simulink model "STP"  (R2021b)
settings: Solver=VariableStepAuto  StartTime=0.0  StopTime=20  RelTol=1e-3
values from neighbouring files (symbols this model uses):
  a0 = mianownik_d(1,4)    [StpProjekt1.m]
  a1 = mianownik_d(1,3)    [StpProjekt1.m]
  a2 = mianownik_d(1,2)    [StpProjekt1.m]
  b0 = licznik_d(1,4)    [StpProjekt1.m]
  b1 = licznik_d(1,3)    [StpProjekt1.m]
  b2 = licznik_d(1,2)    [StpProjekt1.m]
  K_zr = acker(AII,BII,[zb zb zb])    [StpProjekt1.m]
  L1 = acker(A',C', [zo1 zo1 zo1])    [StpProjekt1.m]
  L2 = acker(A',C', [zo2 zo2 zo2])    [StpProjekt1.m]
  L3 = acker(A',C', [zo3 zo3 zo3])    [StpProjekt1.m]
  L4 = acker(A',C', [zo4 zo4 zo4])    [StpProjekt1.m]
  L5 = acker(A',C', [zo5 zo5 zo5])    [StpProjekt1.m]
  T = 0.5    [StpProjekt1.m]
  zb = 0.005    [StpProjekt1.m]
  zb1 = 0.8    [StpProjekt1.m]
  zb2 = 0.4    [StpProjekt1.m]
  zb3 = 0.1    [StpProjekt1.m]
  zb4 = 0.05    [StpProjekt1.m]
  zb5 = 0.005    [StpProjekt1.m]
  zo1 = 0.7    [StpProjekt1.m]
  zo2 = 0.4    [StpProjekt1.m]
  zo3 = 0.25    [StpProjekt1.m]
  zo4 = 0.1    [StpProjekt1.m]
  zo5 = 0.05    [StpProjekt1.m]
settings Model: Creator=Adam  LastModifiedBy=Adam

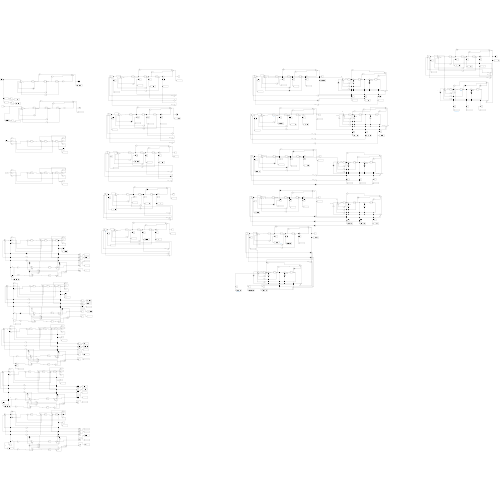
[thumbnail: Simulink's stored preview of the top-level diagram]
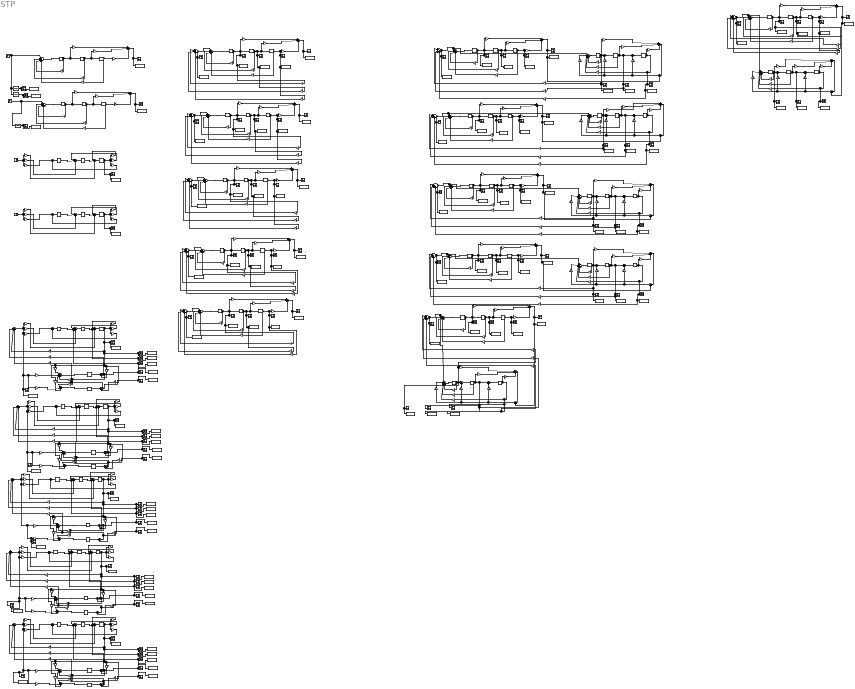
== system STP ==
  note: y(k)
  note: u(k)
  note: u(k)
  note: y(k)
  note: y(k)
  note: u(k)
  note: u(k)
  note: y(k)
  note: u(k)
  note: y(k)
  note: y(k)
  note: u(k)
  note: y(k)
  note: u(k)
  note: y(k)
  note: u(k)
  note: y(k)
  note: u(k)
  note: y(k)
  note: u(k)
  note: u(k)
  note: y(k)
  Delay{,1..5,24..25,29..35,45..47,54..56,82..83,87} (24 alike) : Delay  DelayLength=1  InitialCondition=0  SampleTime=T
  Delay{7,10,19,22,27,37,40,43,49,52,58,63,68,73,78,85} (16 alike) : Delay  DelayLength=1  InitialCondition=-3  SampleTime=T
  Delay{8,11..12,17,20,23,28,38,41,44,50,53,57,62,67,72,77,86} (18 alike) : Delay  DelayLength=1  InitialCondition=1  SampleTime=T
  Delay13 : Delay  DelayLength=1  InitialCondition=2  SampleTime=T
  Delay14 : Delay  DelayLength=1  InitialCondition=3  SampleTime=T
  Delay15 : Delay  DelayLength=1  InitialCondition=3  SampleTime=T
  Delay16 : Delay  DelayLength=1  InitialCondition=2  SampleTime=T
  Delay{6,9,18,21,26,36,39,42,48,51,59,64,69,74,79,84} (16 alike) : Delay  DelayLength=1  InitialCondition=-5  SampleTime=T
  Delay{60..61,65..66,70..71,75..76,80..81} (10 alike) : Delay  DelayLength=1  InitialCondition=0
  Discrete Transfer Fcn : DiscreteTransferFcn  Numerator=[0 0.0104 -8.7322e-04 1.2562e-05]  Denominator=[1 -0.0133 5.4368e-05 -6.8256e-08]  SampleTime=T
  Discrete Transfer Fcn1 : DiscreteTransferFcn  Numerator=[0 0.0104 -8.7322e-04 1.2562e-05]  Denominator=[1 -0.0133 5.4368e-05 -6.8256e-08]  InitialStates=[1 2 3]  SampleTime=T
  Gain{,176,193,210,227} (5 alike) : Gain  Gain=K_zr(1)
  Gain{1,6,13,22,30,38,42,51,60..61,78,87,97,106,114,124,132,141,153,159,179,196,213,230,244..245} (26 alike) : Gain  Gain=b2
  Gain{3,10,16,25,33,36,45,54,64,71,80,89,100,109,117,127,134,144,151,161,177,194,211,228,248,255} (26 alike) : Gain  Gain=-a1
  Gain{4,9,17,26,34,41,46,55,65,70,79,88,101,110,118,128,133,145,156,160,182,199,216,233,249,254} (26 alike) : Gain  Gain=-a2
  Gain{5,8,18,27,35,40,47,56,66,74,83,92,102,111,119,129,137,146,155,164,181,198,215,232,250,258} (26 alike) : Gain  Gain=b0
  Gain{28,67,103,112,130,251} (6 alike) : Gain  Gain=-(-3*zb-a2)
  Gain{29,68,104,113,131,252} (6 alike) : Gain  Gain=-(3*zb^2-a1)
  Gain{69,96,105,123,150,253} (6 alike) : Gain  Gain=-(-zb^3-a0)
  Gain{11..12,14,23,31,37,43,52,62,72,81,90,98,107,115,125,135,142,152,162,178,195,212,229,246,256} (26 alike) : Gain  Gain=-a0
  Gain{2,7,15,24,32,39,44,53,63,73,82,91,99,108,116,126,136,143,154,163,180,197,214,231,247,257} (26 alike) : Gain  Gain=b1
  Gain120 : Gain  Gain=-(-3*zb4-a2)
  Gain121 : Gain  Gain=-(3*zb4^2-a1)
  Gain122 : Gain  Gain=-(-zb4^3-a0)
  Gain138 : Gain  Gain=L4(2)
  Gain139 : Gain  Gain=L4(3)
  Gain140 : Gain  Gain=L4(1)
  Gain147 : Gain  Gain=-(-3*zb5-a2)
  Gain148 : Gain  Gain=-(3*zb5^2-a1)
  Gain149 : Gain  Gain=-(-zb5^3-a0)
  Gain{157,183,200,217,234} (5 alike) : Gain  Gain=K_zr(2)
  Gain{158,184,201,218,235} (5 alike) : Gain  Gain=K_zr(3)
  Gain165 : Gain  Gain=L5(2)
  Gain166 : Gain  Gain=L5(3)
  Gain167 : Gain  Gain=L5(1)
  Gain168 : Gain  Gain=b1+2*b2*zo1
  Gain169 : Gain  Gain=b0-b2*zo1^2
  Gain170 : Gain  Gain=-a1-2*a2*zo1
  Gain171 : Gain  Gain=-a0+a2*zo1^2
  Gain172 : Gain  Gain=-zo1^2
  Gain173 : Gain  Gain=2*zo1
  Gain174 : Gain  Gain=-2*zo1
  Gain175 : Gain  Gain=zo1^2
  Gain185 : Gain  Gain=b1+2*b2*zo2
  Gain186 : Gain  Gain=b0-b2*zo2^2
  Gain187 : Gain  Gain=-a1-2*a2*zo2
  Gain188 : Gain  Gain=-a0+a2*zo2^2
  Gain189 : Gain  Gain=-zo2^2
  Gain19 : Gain  Gain=-(-3*zb1-a2)
  Gain190 : Gain  Gain=2*zo2
  Gain191 : Gain  Gain=-2*zo2
  Gain192 : Gain  Gain=zo2^2
  Gain20 : Gain  Gain=-(3*zb1^2-a1)
  Gain202 : Gain  Gain=b1+2*b2*zo3
  Gain203 : Gain  Gain=b0-b2*zo3^2
  Gain204 : Gain  Gain=-a1-2*a2*zo3
  Gain205 : Gain  Gain=-a0+a2*zo3^2
  Gain206 : Gain  Gain=-zo3^2
  Gain207 : Gain  Gain=2*zo3
  Gain208 : Gain  Gain=-2*zo3
  Gain209 : Gain  Gain=zo3^2
  Gain21 : Gain  Gain=-(-zb1^3-a0)
  Gain219 : Gain  Gain=b1+2*b2*zo4
  Gain220 : Gain  Gain=b0-b2*zo4^2
  Gain221 : Gain  Gain=-a1-2*a2*zo4
  Gain222 : Gain  Gain=-a0+a2*zo4^2
  Gain223 : Gain  Gain=-zo4^2
  Gain224 : Gain  Gain=2*zo4
  Gain225 : Gain  Gain=-2*zo4
  Gain226 : Gain  Gain=zo4^2
  Gain236 : Gain  Gain=b1+2*b2*zo5
  Gain237 : Gain  Gain=b0-b2*zo5^2
  Gain238 : Gain  Gain=-a1-2*a2*zo5
  Gain239 : Gain  Gain=-a0+a2*zo5^2
  Gain240 : Gain  Gain=-zo5^2
  Gain241 : Gain  Gain=2*zo5
  Gain242 : Gain  Gain=-2*zo5
  Gain243 : Gain  Gain=zo5^2
  Gain259 : Gain  Gain=L1(2)
  Gain260 : Gain  Gain=L1(3)
  Gain261 : Gain  Gain=L1(1)
  Gain48 : Gain  Gain=-(-3*zb2-a2)
  Gain49 : Gain  Gain=-(3*zb2^2-a1)
  Gain50 : Gain  Gain=-(-zb2^3-a0)
  Gain57 : Gain  Gain=-(-3*zb3-a2)
  Gain58 : Gain  Gain=-(3*zb3^2-a1)
  Gain59 : Gain  Gain=-(-zb3^3-a0)
  Gain75 : Gain  Gain=L1(2)
  Gain76 : Gain  Gain=L1(3)
  Gain77 : Gain  Gain=L1(1)
  Gain84 : Gain  Gain=L2(2)
  Gain85 : Gain  Gain=L2(3)
  Gain86 : Gain  Gain=L2(1)
  Gain93 : Gain  Gain=L3(2)
  Gain94 : Gain  Gain=L3(3)
  Gain95 : Gain  Gain=L3(1)
  Scope{,1..114} (115 alike) : Scope
  Step{,1..3} (4 alike) : Step  SampleTime=0
  Sum{,5,8,11,13,18,21,27,43,46,48,59,70,78,86,94,102,108} (18 alike) : Sum  Inputs=|++++
  Sum{1,3..4,6..7,9..10,12,14,16..17,19..20,22..23,25,28..29,33,38,42,44..45,47,49..50,52,56,58,60..61,63,67..69,74..77,82..85,90..93,98..101,106,109..110} (54 alike) : Sum  Inputs=|+++
  Sum{2,15,24,31..32,36..37,41,51,55,57,62,66,71..73,79..81,87..89,95..97,103..105,112} (29 alike) : Sum  Inputs=|++
  Sum{26,34,39,53,64,107} (6 alike) : Sum  Inputs=|-+
  Sum{30,35,40,54,65,111} (6 alike) : Sum  Inputs=|+++++
  To Workspace : ToWorkspace  VariableName=dyskretny1_zer  SaveFormat=Structure With Time  SampleTime=-1
  To Workspace1 : ToWorkspace  VariableName=dyskretny2_zer  SaveFormat=Structure With Time  SampleTime=-1
  To Workspace10 : ToWorkspace  VariableName=u_zb_zo2  SaveFormat=Structure With Time  SampleTime=-1
  To Workspace100 : ToWorkspace  VariableName=x2est_zre_zo5  SaveFormat=Structure With Time  SampleTime=-1
  To Workspace101 : ToWorkspace  VariableName=x3est_zre_zo5  SaveFormat=Structure With Time  SampleTime=-1
  To Workspace102 : ToWorkspace  VariableName=u_zre_zo1  SaveFormat=Structure With Time  SampleTime=-1
  To Workspace103 : ToWorkspace  VariableName=u_zre_zo2  SaveFormat=Structure With Time  SampleTime=-1
  To Workspace104 : ToWorkspace  VariableName=u_zre_zo3  SaveFormat=Structure With Time  SampleTime=-1
  To Workspace105 : ToWorkspace  VariableName=u_zre_zo4  SaveFormat=Structure With Time  SampleTime=-1
  To Workspace106 : ToWorkspace  VariableName=u_zre_zo5  SaveFormat=Structure With Time  SampleTime=-1
  To Workspace107 : ToWorkspace  VariableName=x2est_zo  SaveFormat=Structure With Time  SampleTime=-1
  To Workspace108 : ToWorkspace  VariableName=x3est_zo  SaveFormat=Structure With Time  SampleTime=-1
  To Workspace109 : ToWorkspace  VariableName=z_regulatorem10  SaveFormat=Structure With Time  SampleTime=-1
  To Workspace11 : ToWorkspace  VariableName=x1_zb_zo2  SaveFormat=Structure With Time  SampleTime=-1
  To Workspace110 : ToWorkspace  VariableName=u_zb_zo  SaveFormat=Structure With Time  SampleTime=-1
  To Workspace111 : ToWorkspace  VariableName=x1_zb_zo  SaveFormat=Structure With Time  SampleTime=-1
  To Workspace112 : ToWorkspace  VariableName=x2_zb_zo  SaveFormat=Structure With Time  SampleTime=-1
  To Workspace113 : ToWorkspace  VariableName=x3_zb_zo  SaveFormat=Structure With Time  SampleTime=-1
  To Workspace114 : ToWorkspace  VariableName=x1est_zo  SaveFormat=Structure With Time  SampleTime=-1
  To Workspace12 : ToWorkspace  VariableName=dyskretny1_niezer  SaveFormat=Structure With Time  SampleTime=-1
  To Workspace13 : ToWorkspace  VariableName=transm_z_niezer  SaveFormat=Structure With Time  SampleTime=-1
  To Workspace14 : ToWorkspace  VariableName=z_regulatorem1  SaveFormat=Structure With Time  SampleTime=-1
  To Workspace15 : ToWorkspace  VariableName=dyskretny2_niezer  SaveFormat=Structure With Time  SampleTime=-1
  To Workspace16 : ToWorkspace  VariableName=u_zb2  SaveFormat=Structure With Time  SampleTime=-1
  To Workspace17 : ToWorkspace  VariableName=x1_zb2  SaveFormat=Structure With Time  SampleTime=-1
  To Workspace18 : ToWorkspace  VariableName=x2_zb2  SaveFormat=Structure With Time  SampleTime=-1
  To Workspace19 : ToWorkspace  VariableName=x3_zb2  SaveFormat=Structure With Time  SampleTime=-1
  To Workspace2 : ToWorkspace  VariableName=transm_z_zer  SaveFormat=Structure With Time  SampleTime=-1
  To Workspace20 : ToWorkspace  VariableName=z_regulatorem2  SaveFormat=Structure With Time  SampleTime=-1
  To Workspace21 : ToWorkspace  VariableName=u_zb3  SaveFormat=Structure With Time  SampleTime=-1
  To Workspace22 : ToWorkspace  VariableName=x1_zb3  SaveFormat=Structure With Time  SampleTime=-1
  To Workspace23 : ToWorkspace  VariableName=x2_zb3  SaveFormat=Structure With Time  SampleTime=-1
  To Workspace24 : ToWorkspace  VariableName=x3_zb3  SaveFormat=Structure With Time  SampleTime=-1
  To Workspace25 : ToWorkspace  VariableName=x2est_zo1  SaveFormat=Structure With Time  SampleTime=-1
  To Workspace26 : ToWorkspace  VariableName=x3est_zo1  SaveFormat=Structure With Time  SampleTime=-1
  To Workspace27 : ToWorkspace  VariableName=z_regulatorem3  SaveFormat=Structure With Time  SampleTime=-1
  To Workspace28 : ToWorkspace  VariableName=u_zb_zo1  SaveFormat=Structure With Time  SampleTime=-1
  To Workspace29 : ToWorkspace  VariableName=x1_zb_zo1  SaveFormat=Structure With Time  SampleTime=-1
  To Workspace3 : ToWorkspace  VariableName=z_regulatorem6  SaveFormat=Structure With Time  SampleTime=-1
  To Workspace30 : ToWorkspace  VariableName=x2_zb_zo1  SaveFormat=Structure With Time  SampleTime=-1
  To Workspace31 : ToWorkspace  VariableName=x3_zb_zo1  SaveFormat=Structure With Time  SampleTime=-1
  To Workspace32 : ToWorkspace  VariableName=x1est_zo1  SaveFormat=Structure With Time  SampleTime=-1
  To Workspace33 : ToWorkspace  VariableName=x2est_zo2  SaveFormat=Structure With Time  SampleTime=-1
  To Workspace34 : ToWorkspace  VariableName=x3est_zo2  SaveFormat=Structure With Time  SampleTime=-1
  To Workspace35 : ToWorkspace  VariableName=x1est_zo2  SaveFormat=Structure With Time  SampleTime=-1
  To Workspace36 : ToWorkspace  VariableName=x2est_zo3  SaveFormat=Structure With Time  SampleTime=-1
  To Workspace37 : ToWorkspace  VariableName=x3est_zo3  SaveFormat=Structure With Time  SampleTime=-1
  To Workspace38 : ToWorkspace  VariableName=x1est_zo3  SaveFormat=Structure With Time  SampleTime=-1
  To Workspace39 : ToWorkspace  VariableName=x2_zb_zo2  SaveFormat=Structure With Time  SampleTime=-1
  To Workspace4 : ToWorkspace  VariableName=z_regulatorem  SaveFormat=Structure With Time  SampleTime=-1
  To Workspace40 : ToWorkspace  VariableName=x3_zb_zo2  SaveFormat=Structure With Time  SampleTime=-1
  To Workspace41 : ToWorkspace  VariableName=z_regulatorem5  SaveFormat=Structure With Time  SampleTime=-1
  To Workspace42 : ToWorkspace  VariableName=u_zb_zo3  SaveFormat=Structure With Time  SampleTime=-1
  To Workspace43 : ToWorkspace  VariableName=x1_zb_zo3  SaveFormat=Structure With Time  SampleTime=-1
  To Workspace44 : ToWorkspace  VariableName=x2_zb_zo3  SaveFormat=Structure With Time  SampleTime=-1
  To Workspace45 : ToWorkspace  VariableName=x3_zb_zo3  SaveFormat=Structure With Time  SampleTime=-1
  To Workspace46 : ToWorkspace  VariableName=z_regulatorem7  SaveFormat=Structure With Time  SampleTime=-1
  To Workspace47 : ToWorkspace  VariableName=u_zb_zo4  SaveFormat=Structure With Time  SampleTime=-1
  To Workspace48 : ToWorkspace  VariableName=x1_zb_zo4  SaveFormat=Structure With Time  SampleTime=-1
  To Workspace49 : ToWorkspace  VariableName=u_zb4  SaveFormat=Structure With Time  SampleTime=-1
  To Workspace5 : ToWorkspace  VariableName=u_zb1  SaveFormat=Structure With Time  SampleTime=-1
  To Workspace50 : ToWorkspace  VariableName=x1_zb4  SaveFormat=Structure With Time  SampleTime=-1
  To Workspace51 : ToWorkspace  VariableName=x2_zb4  SaveFormat=Structure With Time  SampleTime=-1
  To Workspace52 : ToWorkspace  VariableName=x3_zb4  SaveFormat=Structure With Time  SampleTime=-1
  To Workspace53 : ToWorkspace  VariableName=x2est_zo4  SaveFormat=Structure With Time  SampleTime=-1
  To Workspace54 : ToWorkspace  VariableName=x3est_zo4  SaveFormat=Structure With Time  SampleTime=-1
  To Workspace55 : ToWorkspace  VariableName=x1est_zo4  SaveFormat=Structure With Time  SampleTime=-1
  To Workspace56 : ToWorkspace  VariableName=x2_zb_zo4  SaveFormat=Structure With Time  SampleTime=-1
  To Workspace57 : ToWorkspace  VariableName=x3_zb_zo4  SaveFormat=Structure With Time  SampleTime=-1
  To Workspace58 : ToWorkspace  VariableName=z_regulatorem9  SaveFormat=Structure With Time  SampleTime=-1
  To Workspace59 : ToWorkspace  VariableName=u_zb_zo5  SaveFormat=Structure With Time  SampleTime=-1
  To Workspace6 : ToWorkspace  VariableName=x1_zb1  SaveFormat=Structure With Time  SampleTime=-1
  To Workspace60 : ToWorkspace  VariableName=x1_zb_zo5  SaveFormat=Structure With Time  SampleTime=-1
  To Workspace61 : ToWorkspace  VariableName=transm_s  SaveFormat=Structure With Time  SampleTime=-1
  To Workspace62 : ToWorkspace  VariableName=z_regulatorem8  SaveFormat=Structure With Time  SampleTime=-1
  To Workspace63 : ToWorkspace  VariableName=u_zb5  SaveFormat=Structure With Time  SampleTime=-1
  To Workspace64 : ToWorkspace  VariableName=x1_zb5  SaveFormat=Structure With Time  SampleTime=-1
  To Workspace65 : ToWorkspace  VariableName=x2_zb5  SaveFormat=Structure With Time  SampleTime=-1
  To Workspace66 : ToWorkspace  VariableName=x3_zb5  SaveFormat=Structure With Time  SampleTime=-1
  To Workspace67 : ToWorkspace  VariableName=x2est_zo5  SaveFormat=Structure With Time  SampleTime=-1
  To Workspace68 : ToWorkspace  VariableName=x3est_zo5  SaveFormat=Structure With Time  SampleTime=-1
  To Workspace69 : ToWorkspace  VariableName=x1est_zo5  SaveFormat=Structure With Time  SampleTime=-1
  To Workspace7 : ToWorkspace  VariableName=x2_zb1  SaveFormat=Structure With Time  SampleTime=-1
  To Workspace70 : ToWorkspace  VariableName=x2_zb_zo5  SaveFormat=Structure With Time  SampleTime=-1
  To Workspace71 : ToWorkspace  VariableName=x3_zb_zo5  SaveFormat=Structure With Time  SampleTime=-1
  To Workspace72 : ToWorkspace  VariableName=dyskretny2_niezer1  SaveFormat=Structure With Time  SampleTime=-1
  To Workspace73 : ToWorkspace  VariableName=x1zre_zo1  SaveFormat=Structure With Time  SampleTime=-1
  To Workspace74 : ToWorkspace  VariableName=x2zre_zo1  SaveFormat=Structure With Time  SampleTime=-1
  To Workspace75 : ToWorkspace  VariableName=x3zre_zo1  SaveFormat=Structure With Time  SampleTime=-1
  To Workspace76 : ToWorkspace  VariableName=x2est_zre_zo1  SaveFormat=Structure With Time  SampleTime=-1
  To Workspace77 : ToWorkspace  VariableName=x3est_zre_zo1  SaveFormat=Structure With Time  SampleTime=-1
  To Workspace78 : ToWorkspace  VariableName=dyskretny2_niezer2  SaveFormat=Structure With Time  SampleTime=-1
  To Workspace79 : ToWorkspace  VariableName=x1zre_zo2  SaveFormat=Structure With Time  SampleTime=-1
  To Workspace8 : ToWorkspace  VariableName=x3_zb1  SaveFormat=Structure With Time  SampleTime=-1
  To Workspace80 : ToWorkspace  VariableName=x2zre_zo2  SaveFormat=Structure With Time  SampleTime=-1
  To Workspace81 : ToWorkspace  VariableName=x3zre_zo2  SaveFormat=Structure With Time  SampleTime=-1
  To Workspace82 : ToWorkspace  VariableName=x2est_zre_zo2  SaveFormat=Structure With Time  SampleTime=-1
  To Workspace83 : ToWorkspace  VariableName=x3est_zre_zo2  SaveFormat=Structure With Time  SampleTime=-1
  To Workspace84 : ToWorkspace  VariableName=dyskretny2_niezer3  SaveFormat=Structure With Time  SampleTime=-1
  To Workspace85 : ToWorkspace  VariableName=x1zre_zo3  SaveFormat=Structure With Time  SampleTime=-1
  To Workspace86 : ToWorkspace  VariableName=x2zre_zo3  SaveFormat=Structure With Time  SampleTime=-1
  To Workspace87 : ToWorkspace  VariableName=x3zre_zo3  SaveFormat=Structure With Time  SampleTime=-1
  To Workspace88 : ToWorkspace  VariableName=x2est_zre_zo3  SaveFormat=Structure With Time  SampleTime=-1
  To Workspace89 : ToWorkspace  VariableName=x3est_zre_zo3  SaveFormat=Structure With Time  SampleTime=-1
  To Workspace9 : ToWorkspace  VariableName=z_regulatorem4  SaveFormat=Structure With Time  SampleTime=-1
  To Workspace90 : ToWorkspace  VariableName=dyskretny2_niezer4  SaveFormat=Structure With Time  SampleTime=-1
  To Workspace91 : ToWorkspace  VariableName=x1zre_zo4  SaveFormat=Structure With Time  SampleTime=-1
  To Workspace92 : ToWorkspace  VariableName=x2zre_zo4  SaveFormat=Structure With Time  SampleTime=-1
  To Workspace93 : ToWorkspace  VariableName=x3zre_zo4  SaveFormat=Structure With Time  SampleTime=-1
  To Workspace94 : ToWorkspace  VariableName=x2est_zre_zo4  SaveFormat=Structure With Time  SampleTime=-1
  To Workspace95 : ToWorkspace  VariableName=x3est_zre_zo4  SaveFormat=Structure With Time  SampleTime=-1
  To Workspace96 : ToWorkspace  VariableName=dyskretny2_niezer5  SaveFormat=Structure With Time  SampleTime=-1
  To Workspace97 : ToWorkspace  VariableName=x1zre_zo5  SaveFormat=Structure With Time  SampleTime=-1
  To Workspace98 : ToWorkspace  VariableName=x2zre_zo5  SaveFormat=Structure With Time  SampleTime=-1
  To Workspace99 : ToWorkspace  VariableName=x3zre_zo5  SaveFormat=Structure With Time  SampleTime=-1
  Transfer Fcn : TransferFcn  Numerator=[1 10 12.75]  Denominator=[1 33 362 1320]
  wires:
  Sum/1 -> Delay/1  "x1(k+1) E(z)"
  Delay/1 -> Gain4/1, Gain1/1, Delay1/1  "x2(k+1)=x1(k) (z^-1)E(z)"
  Delay1/1 -> Gain2/1, Delay2/1, Gain3/1  "x3(k+1)=x2(k) (z^-2)E(z)"
  Sum1/1 -> To Workspace/1, Scope/1  "y(k) Y(z)"
  Step/1 -> Transfer Fcn/1, Discrete Transfer Fcn/1, Sum/1  "u(k) U(z)"
  Gain1/1 -> Sum1/1
  Gain4/1 -> Sum/3
  Gain3/1 -> Sum/2
  Gain2/1 -> Sum1/2
  Delay2/1 -> Gain12/1, Gain5/1  "x3(k) (z^-3)E(z)"
  Gain12/1 -> Sum/4
  Gain5/1 -> Sum1/3
  Sum2/1 -> Delay3/1  "x3(k+1)"
  Sum3/1 -> Delay4/1  "x2(k+1)"
  Sum4/1 -> Delay5/1  "x1(k+1)"
  Delay5/1 -> To Workspace1/1, Scope1/1, Gain11/1, Gain10/1, Gain9/1  "y(k)=x1(k)"
  Step1/1 -> Gain8/1, Gain6/1, Gain7/1  "u(k)"
  Gain8/1 -> Sum2/1
  Gain11/1 -> Sum2/2
  Delay3/1 -> Sum3/2  "x3(k)"
  Gain7/1 -> Sum3/3
  Gain10/1 -> Sum3/1
  Gain9/1 -> Sum4/1
  Delay4/1 -> Sum4/2  "x2(k)"
  Gain6/1 -> Sum4/3
  Discrete Transfer Fcn/1 -> To Workspace2/1, Scope2/1
  Gain16/1 -> Sum5/2
  Delay6/1 -> Gain17/1, Gain13/1, Delay7/1, Gain19/1, To Workspace6/1, Scope5/1  "x2(k+1)=x1(k) (z^-1)E(z)"
  Delay7/1 -> Gain20/1, To Workspace7/1, Scope6/1, Gain15/1, Delay8/1, Gain16/1  "x3(k+1)=x2(k) (z^-2)E(z)"
  Gain17/1 -> Sum5/3
  Gain14/1 -> Sum5/4
  Gain13/1 -> Sum6/1
  Sum6/1 -> To Workspace4/1, Scope4/1  "y(k) Y(z)"
  Gain18/1 -> Sum6/3
  Gain15/1 -> Sum6/2
  Sum5/1 -> Delay6/1  "x1(k+1) E(z)"
  Delay8/1 -> Gain14/1, Gain21/1, To Workspace8/1, Scope7/1, Gain18/1  "x3(k) (z^-3)E(z)"
  Sum7/1 -> To Workspace5/1, Scope8/1, Sum5/1  "u(k)"
  Gain19/1 -> Sum7/1  "-k1x1(k)"
  Gain20/1 -> Sum7/2  "-k2x2(k)"
  Gain21/1 -> Sum7/3  "-k3x3(k)"
  Sum13/1 -> Delay12/1  "x1(k+1) E(z)"
  Sum14/1 -> To Workspace12/1, Scope12/1  "y(k) Y(z)"
  Gain35/1 -> Sum14/3
  Step2/1 -> Discrete Transfer Fcn1/1, Sum13/1  "u(k) U(z)"
  Gain30/1 -> Sum14/1
  Discrete Transfer Fcn1/1 -> To Workspace13/1, Scope13/1
  Delay14/1 -> Gain31/1, Gain35/1  "x3(k) (z^-3)E(z)"
  Delay13/1 -> Gain32/1, Delay14/1, Gain33/1  "x3(k+1)=x2(k) (z^-2)E(z)"
  Gain32/1 -> Sum14/2
  Gain31/1 -> Sum13/4
  Delay12/1 -> Gain34/1, Gain30/1, Delay13/1  "x2(k+1)=x1(k) (z^-1)E(z)"
  Gain34/1 -> Sum13/3
  Gain33/1 -> Sum13/2
  Sum17/1 -> Delay17/1  "x1(k+1)"
  Delay16/1 -> Sum17/2  "x2(k)"
  Gain41/1 -> Sum17/1
  Step3/1 -> Gain40/1, Gain38/1, Gain39/1  "u(k)"
  Sum16/1 -> Delay16/1  "x2(k+1)"
  Delay17/1 -> To Workspace15/1, Scope15/1, Gain37/1, Gain36/1, Gain41/1  "y(k)=x1(k)"
  Gain38/1 -> Sum17/3
  Sum15/1 -> Delay15/1  "x3(k+1)"
  Gain36/1 -> Sum16/1
  Gain39/1 -> Sum16/3
  Gain40/1 -> Sum15/1
  Gain37/1 -> Sum15/2
  Delay15/1 -> Sum16/2  "x3(k)"
  Gain50/1 -> Sum20/3  "-k3x3(k)"
  Gain47/1 -> Sum19/3
  Gain42/1 -> Sum19/1
  Gain44/1 -> Sum19/2
  Gain49/1 -> Sum20/2  "-k2x2(k)"
  Delay19/1 -> Gain49/1, To Workspace18/1, Scope17/1, Gain44/1, Delay20/1, Gain45/1  "x3(k+1)=x2(k) (z^-2)E(z)"
  Delay18/1 -> Gain46/1, Gain42/1, Delay19/1, Gain48/1, To Workspace17/1, Scope16/1  "x2(k+1)=x1(k) (z^-1)E(z)"
  Sum18/1 -> Delay18/1  "x1(k+1) E(z)"
  Gain46/1 -> Sum18/3
  Sum19/1 -> To Workspace14/1, Scope14/1  "y(k) Y(z)"
  Gain43/1 -> Sum18/4
  Gain45/1 -> Sum18/2
  Delay20/1 -> Gain43/1, Gain50/1, To Workspace19/1, Scope18/1, Gain47/1  "x3(k) (z^-3)E(z)"
  Gain48/1 -> Sum20/1  "-k1x1(k)"
  Sum20/1 -> To Workspace16/1, Scope19/1, Sum18/1  "u(k)"
  Sum21/1 -> Delay21/1  "x1(k+1) (z)"
  Delay21/1 -> Gain55/1, Gain51/1, Delay22/1, Gain57/1, To Workspace22/1, Scope21/1  "x2(k+1)=x1(k) (z^-1)E(z)"
  Delay22/1 -> Gain58/1, To Workspace23/1, Scope22/1, Gain53/1, Delay23/1, Gain54/1  "x3(k+1)=x2(k) (z^-2)E(z)"
  Sum23/1 -> To Workspace21/1, Scope24/1, Sum21/1  "u(k)"
  Gain55/1 -> Sum21/3
  Delay23/1 -> Gain52/1, Gain59/1, To Workspace24/1, Scope23/1, Gain56/1  "x3(k) (z^-3)E(z)"
  Gain54/1 -> Sum21/2
  Gain52/1 -> Sum21/4
  Sum22/1 -> To Workspace20/1, Scope20/1  "y(k)"
  Gain53/1 -> Sum22/2
  Gain58/1 -> Sum23/2  "-k2x2(k)"
  Gain51/1 -> Sum22/1
  Gain56/1 -> Sum22/3
  Gain59/1 -> Sum23/3  "-k3x3(k)"
  Gain57/1 -> Sum23/1  "-k1x1(k)"
  Delay28/1 -> Gain62/1, To Workspace31/1, Scope30/1, Gain66/1  "x3(k) (z^-3)E(z)"
  Gain68/1 -> Sum29/2  "-k2x2(k)"
  Gain75/1 -> Sum31/2  "l2(y(k)-yest(k))"
  Gain60/1 -> Sum25/1
  Sum26/1 -> Gain76/1, Gain75/1, Gain77/1  "(y(k)-yest(k))"
  Delay24/1 -> Gain71/1, Gain73/1, To Workspace25/1, Gain68/1, Scope25/1, Sum24/1  "x2est(k)"
  Delay25/1 -> Gain74/1, Gain69/1, To Workspace26/1, Scope26/1, Gain72/1  "x3est(k)"
  Gain76/1 -> Sum24/2  "l3(y(k)-yest(k))"
  Gain77/1 -> Sum30/2  "l1(y(k)-yest(k))"
  Gain66/1 -> Sum28/3
  Gain61/1 -> Sum28/1
  Gain63/1 -> Sum28/2
  Delay27/1 -> To Workspace30/1, Scope29/1, Gain63/1, Delay28/1, Gain64/1  "x3(k+1)=x2(k) (z^-2)E(z)"
  Delay26/1 -> Gain65/1, Gain61/1, Delay27/1, To Workspace29/1, Scope28/1  "x2(k+1)=x1(k) (z^-1)E(z)"
  Sum27/1 -> Delay26/1  "x1(k+1) E(z)"
  Gain71/1 -> Sum30/4
  Sum24/1 -> Delay25/1  "x3est(k+1)"
  Sum25/1 -> Sum26/1  "yest(k)"
  Gain65/1 -> Sum27/3
  Gain62/1 -> Sum27/4
  Gain73/1 -> Sum25/2
  Gain67/1 -> Sum29/1  "-k1x1(k)"
  Gain70/1 -> Sum30/5
  Gain64/1 -> Sum27/2
  Delay29/1 -> Gain70/1, Gain60/1, Sum31/1, To Workspace32/1, Scope32/1, Gain67/1  "x1est(k)"
  Gain69/1 -> Sum29/3  "-k3x3(k)"
  Sum31/1 -> Delay24/1  "x2est(k+1)"
  Gain72/1 -> Sum30/3
  Sum29/1 -> To Workspace28/1, Scope31/1, Sum30/1, Sum27/1  "u(k)"
  Sum30/1 -> Delay29/1  "x1est(k+1)"
  Gain74/1 -> Sum25/3
  Delay30/1 -> Gain80/1, Gain82/1, Gain29/1, To Workspace33/1, Scope33/1, Sum32/1  "x2est(k)"
  Sum34/1 -> Gain85/1, Gain84/1, Gain86/1  "(y(k)-yest(k))"
  Gain84/1 -> Sum36/2  "l2(y(k)-yest(k))"
  Delay31/1 -> Gain83/1, Gain96/1, To Workspace34/1, Scope34/1, Gain81/1  "x3est(k)"
  Gain78/1 -> Sum33/1
  Delay32/1 -> Gain79/1, Gain78/1, Sum36/1, Gain28/1, To Workspace35/1, Scope35/1  "x1est(k)"
  Sum36/1 -> Delay30/1  "x2est(k+1)"
  Gain79/1 -> Sum35/5
  Gain82/1 -> Sum33/2
  Sum28/1 -> To Workspace27/1, Sum26/2, Scope27/1  "y(k) Y(z)"
  Sum33/1 -> Sum34/1  "yest(k)"
  Gain83/1 -> Sum33/3
  Gain85/1 -> Sum32/2  "l3(y(k)-yest(k))"
  Sum35/1 -> Delay32/1  "x1est(k+1)"
  Sum32/1 -> Delay31/1  "x3est(k+1)"
  Gain86/1 -> Sum35/2  "l1(y(k)-yest(k))"
  Gain80/1 -> Sum35/4
  Gain81/1 -> Sum35/3
  Gain90/1 -> Sum40/3
  Gain95/1 -> Sum40/2  "l1(y(k)-yest(k))"
  Gain92/1 -> Sum38/3
  Gain94/1 -> Sum37/2  "l3(y(k)-yest(k))"
  Sum41/1 -> Delay33/1  "x2est(k+1)"
  Gain91/1 -> Sum38/2
  Delay35/1 -> Gain88/1, Gain87/1, Sum41/1, To Workspace38/1, Scope38/1, Gain103/1  "x1est(k)"
  Sum38/1 -> Sum39/1  "yest(k)"
  Gain87/1 -> Sum38/1
  Sum37/1 -> Delay34/1  "x3est(k+1)"
  Sum39/1 -> Gain94/1, Gain93/1, Gain95/1  "(y(k)-yest(k))"
  Gain88/1 -> Sum40/5
  Gain89/1 -> Sum40/4
  Gain93/1 -> Sum41/2  "l2(y(k)-yest(k))"
  Delay33/1 -> Gain89/1, Gain91/1, Gain104/1, To Workspace36/1, Scope36/1, Sum37/1  "x2est(k)"
  Delay34/1 -> Gain92/1, Gain105/1, To Workspace37/1, Scope37/1, Gain90/1  "x3est(k)"
  Sum40/1 -> Delay35/1  "x1est(k+1)"
  Delay44/1 -> Gain115/1, Gain122/1, To Workspace52/1, Scope51/1, Gain119/1  "x3(k) (z^-3)E(z)"
  Gain122/1 -> Sum50/3  "-k3x3(k)"
  Delay43/1 -> Gain121/1, To Workspace51/1, Scope50/1, Gain116/1, Delay44/1, Gain117/1  "x3(k+1)=x2(k) (z^-2)E(z)"
  Gain121/1 -> Sum50/2  "-k2x2(k)"
  Gain114/1 -> Sum49/1
  Gain120/1 -> Sum50/1  "-k1x1(k)"
  Gain118/1 -> Sum48/3
  Gain116/1 -> Sum49/2
  Sum49/1 -> To Workspace3/1, Scope3/1  "y(k)"
  Gain117/1 -> Sum48/2
  Delay42/1 -> Gain118/1, Gain114/1, Delay43/1, Gain120/1, To Workspace50/1, Scope49/1  "x2(k+1)=x1(k) (z^-1)E(z)"
  Gain119/1 -> Sum49/3
  Sum50/1 -> To Workspace49/1, Scope52/1, Sum48/1  "u(k)"
  Sum48/1 -> Delay42/1  "x1(k+1) (z)"
  Gain115/1 -> Sum48/4
  Sum53/1 -> Gain139/1, Gain138/1, Gain140/1  "(y(k)-yest(k))"
  Gain139/1 -> Sum51/2  "l3(y(k)-yest(k))"
  Delay46/1 -> Gain137/1, Gain123/1, To Workspace54/1, Scope54/1, Gain135/1  "x3est(k)"
  Gain133/1 -> Sum54/5
  Gain132/1 -> Sum52/1
  Sum55/1 -> Delay45/1  "x2est(k+1)"
  Gain135/1 -> Sum54/3
  Delay45/1 -> Gain134/1, Gain136/1, To Workspace53/1, Gain113/1, Scope53/1, Sum51/1  "x2est(k)"
  Gain138/1 -> Sum55/2  "l2(y(k)-yest(k))"
  Sum54/1 -> Delay47/1  "x1est(k+1)"
  Delay47/1 -> Gain133/1, Gain132/1, Sum55/1, To Workspace55/1, Scope55/1, Gain112/1  "x1est(k)"
  Gain136/1 -> Sum52/2
  Gain134/1 -> Sum54/4
  Sum52/1 -> Sum53/1  "yest(k)"
  Sum51/1 -> Delay46/1  "x3est(k+1)"
  Gain140/1 -> Sum54/2  "l1(y(k)-yest(k))"
  Gain137/1 -> Sum52/3
  Transfer Fcn/1 -> To Workspace61/1, Scope61/1
  Gain144/1 -> Sum59/2
  Gain148/1 -> Sum61/2  "-k2x2(k)"
  Gain147/1 -> Sum61/1  "-k1x1(k)"
  Gain145/1 -> Sum59/3
  Gain142/1 -> Sum59/4
  Sum59/1 -> Delay51/1  "x1(k+1) (z)"
  Sum61/1 -> To Workspace63/1, Scope66/1, Sum59/1  "u(k)"
  Sum60/1 -> To Workspace62/1, Scope62/1  "y(k)"
  Gain146/1 -> Sum60/3
  Delay51/1 -> Gain145/1, Gain141/1, Delay52/1, Gain147/1, To Workspace64/1, Scope63/1  "x2(k+1)=x1(k) (z^-1)E(z)"
  Gain141/1 -> Sum60/1
  Gain143/1 -> Sum60/2
  Delay52/1 -> Gain148/1, To Workspace65/1, Scope64/1, Gain143/1, Delay53/1, Gain144/1  "x3(k+1)=x2(k) (z^-2)E(z)"
  Delay53/1 -> Gain142/1, Gain149/1, To Workspace66/1, Scope65/1, Gain146/1  "x3(k) (z^-3)E(z)"
  Gain149/1 -> Sum61/3  "-k3x3(k)"
  Gain164/1 -> Sum63/3
  Sum62/1 -> Delay55/1  "x3est(k+1)"
  Sum63/1 -> Sum64/1  "yest(k)"
  Gain167/1 -> Sum65/2  "l1(y(k)-yest(k))"
  Gain163/1 -> Sum63/2
  Gain161/1 -> Sum65/4
  Delay56/1 -> Gain160/1, Gain130/1, Gain159/1, To Workspace69/1, Scope69/1, Sum66/1  "x1est(k)"
  Sum65/1 -> Delay56/1  "x1est(k+1)"
  Delay54/1 -> Gain161/1, Gain163/1, To Workspace67/1, Gain131/1, Scope67/1, Sum62/1  "x2est(k)"
  Sum66/1 -> Delay54/1  "x2est(k+1)"
  Gain159/1 -> Sum63/1
  Gain166/1 -> Sum62/2  "l3(y(k)-yest(k))"
  Delay55/1 -> Gain164/1, To Workspace68/1, Gain150/1, Scope68/1, Gain162/1  "x3est(k)"
  Gain162/1 -> Sum65/3
  Sum64/1 -> Gain166/1, Gain165/1, Gain167/1  "(y(k)-yest(k))"
  Gain160/1 -> Sum65/5
  Gain165/1 -> Sum66/2  "l2(y(k)-yest(k))"
  Sum8/1 -> Delay9/1  "x1(k+1) E(z)"
  Sum10/1 -> To Workspace10/1, Scope40/1, Sum35/1, Sum8/1  "u(k)"
  Delay11/1 -> Gain23/1, To Workspace40/1, Scope39/1, Gain27/1  "x3(k) (z^-3)E(z)"
  Gain22/1 -> Sum9/1
  Sum9/1 -> To Workspace9/1, Sum34/2, Scope9/1  "y(k) Y(z)"
  Gain96/1 -> Sum10/3  "-k3x3(k)"
  Gain28/1 -> Sum10/1  "-k1x1(k)"
  Gain27/1 -> Sum9/3
  Delay9/1 -> Gain26/1, Gain22/1, Delay10/1, To Workspace11/1, Scope10/1  "x2(k+1)=x1(k) (z^-1)E(z)"
  Delay10/1 -> To Workspace39/1, Scope11/1, Gain24/1, Delay11/1, Gain25/1  "x3(k+1)=x2(k) (z^-2)E(z)"
  Gain25/1 -> Sum8/2
  Gain23/1 -> Sum8/4
  Gain29/1 -> Sum10/2  "-k2x2(k)"
  Gain24/1 -> Sum9/2
  Gain26/1 -> Sum8/3
  Sum11/1 -> Delay36/1  "x1(k+1) E(z)"
  Sum42/1 -> To Workspace42/1, Scope45/1, Sum40/1, Sum11/1  "u(k)"
  Delay38/1 -> Gain98/1, To Workspace45/1, Scope44/1, Gain102/1  "x3(k) (z^-3)E(z)"
  Gain97/1 -> Sum12/1
  Sum12/1 -> Sum39/2, To Workspace41/1, Scope41/1  "y(k) Y(z)"
  Gain105/1 -> Sum42/3  "-k3x3(k)"
  Gain103/1 -> Sum42/1  "-k1x1(k)"
  Gain102/1 -> Sum12/3
  Delay36/1 -> Gain101/1, Gain97/1, Delay37/1, To Workspace43/1, Scope42/1  "x2(k+1)=x1(k) (z^-1)E(z)"
  Delay37/1 -> To Workspace44/1, Scope43/1, Gain99/1, Delay38/1, Gain100/1  "x3(k+1)=x2(k) (z^-2)E(z)"
  Gain100/1 -> Sum11/2
  Gain98/1 -> Sum11/4
  Gain104/1 -> Sum42/2  "-k2x2(k)"
  Gain99/1 -> Sum12/2
  Gain101/1 -> Sum11/3
  Sum43/1 -> Delay39/1  "x1(k+1) E(z)"
  Sum45/1 -> To Workspace47/1, Scope57/1, Sum54/1, Sum43/1  "u(k)"
  Delay41/1 -> Gain107/1, To Workspace57/1, Scope56/1, Gain111/1  "x3(k) (z^-3)E(z)"
  Gain106/1 -> Sum44/1
  Sum44/1 -> Sum53/2, To Workspace46/1, Scope46/1  "y(k) Y(z)"
  Gain123/1 -> Sum45/3  "-k3x3(k)"
  Gain112/1 -> Sum45/1  "-k1x1(k)"
  Gain111/1 -> Sum44/3
  Delay39/1 -> Gain110/1, Gain106/1, Delay40/1, To Workspace48/1, Scope47/1  "x2(k+1)=x1(k) (z^-1)E(z)"
  Delay40/1 -> To Workspace56/1, Scope48/1, Gain108/1, Delay41/1, Gain109/1  "x3(k+1)=x2(k) (z^-2)E(z)"
  Gain109/1 -> Sum43/2
  Gain107/1 -> Sum43/4
  Gain113/1 -> Sum45/2  "-k2x2(k)"
  Gain108/1 -> Sum44/2
  Gain110/1 -> Sum43/3
  Sum46/1 -> Delay48/1  "x1(k+1) E(z)"
  Sum56/1 -> To Workspace59/1, Scope71/1, Sum65/1, Sum46/1  "u(k)"
  Delay50/1 -> Gain125/1, To Workspace71/1, Scope70/1, Gain129/1  "x3(k) (z^-3)E(z)"
  Gain124/1 -> Sum47/1
  Sum47/1 -> Sum64/2, To Workspace58/1, Scope58/1  "(k) Y(z)"
  Gain150/1 -> Sum56/3  "-k3x3(k)"
  Gain130/1 -> Sum56/1  "-k1x1(k)"
  Gain129/1 -> Sum47/3
  Delay48/1 -> Gain128/1, Gain124/1, Delay49/1, To Workspace60/1, Scope59/1  "x2(k+1)=x1(k) (z^-1)E(z)"
  Delay49/1 -> To Workspace70/1, Scope60/1, Gain126/1, Delay50/1, Gain127/1  "x3(k+1)=x2(k) (z^-2)E(z)"
  Gain127/1 -> Sum46/2
  Gain125/1 -> Sum46/4
  Gain131/1 -> Sum56/2  "-k2x2(k)"
  Gain126/1 -> Sum47/2
  Gain128/1 -> Sum46/3
  Gain155/1 -> Sum57/1
  Gain156/1 -> Sum67/1
  Delay59/1 -> To Workspace73/1, Scope73/1, Gain175/1, Gain174/1, Gain171/1, Gain170/1, Gain/1, To Workspace72/1, Scope72/1, Gain152/1, Gain151/1, Gain156/1  "y(k)=x1(k)"
  Delay57/1 -> To Workspace75/1, Scope75/1, Sum58/2  "x3(k)"
  Gain153/1 -> Sum67/3
  Sum68/1 -> Gain155/1, To Workspace102/1, Scope102/1, Gain169/1, Gain168/1, Gain153/1, Gain154/1  "u(k)"
  Sum58/1 -> Delay58/1  "x2(k+1)"
  Sum67/1 -> Delay59/1  "x1(k+1)"
  Gain154/1 -> Sum58/3
  Gain151/1 -> Sum58/1
  Delay58/1 -> To Workspace74/1, Scope74/1, Sum67/2  "x2(k)"
  Sum57/1 -> Delay57/1  "x3(k+1)"
  Gain152/1 -> Sum57/2
  Gain/1 -> Sum68/1
  Gain157/1 -> Sum68/2
  Gain158/1 -> Sum68/3
  Gain168/1 -> Sum70/2
  Gain169/1 -> Sum69/2
  Gain170/1 -> Sum70/1
  Gain171/1 -> Sum69/3
  Delay61/1 -> Sum72/1  "z2(k)"
  Gain173/1 -> Sum70/4
  Sum71/1 -> Gain157/1, To Workspace76/1, Scope76/1, Gain172/1, Gain173/1  "w1(k)"
  Sum72/1 -> Gain158/1, Sum70/3, To Workspace77/1, Scope77/1  "w2(k)"
  Delay60/1 -> Sum71/1  "z1(k)"
  Sum69/1 -> Delay61/1  "z2(k+1)"
  Sum70/1 -> Delay60/1  "z1(k+1)"
  Gain172/1 -> Sum69/1
  Gain175/1 -> Sum72/2
  Gain174/1 -> Sum71/2
  Sum79/1 -> Gain183/1, To Workspace82/1, Scope82/1, Gain189/1, Gain190/1  "w1(k)"
  Gain176/1 -> Sum76/1
  Gain184/1 -> Sum76/3
  Gain183/1 -> Sum76/2
  Sum73/1 -> Delay62/1  "x3(k+1)"
  Delay63/1 -> To Workspace80/1, Scope80/1, Sum75/2  "x2(k)"
  Gain190/1 -> Sum78/4
  Sum74/1 -> Delay63/1  "x2(k+1)"
  Gain180/1 -> Sum74/3
  Sum75/1 -> Delay64/1  "x1(k+1)"
  Gain192/1 -> Sum80/2
  Delay62/1 -> To Workspace81/1, Scope81/1, Sum74/2  "x3(k)"
  Delay64/1 -> To Workspace79/1, Scope79/1, Gain192/1, Gain191/1, Gain188/1, Gain187/1, Gain176/1, To Workspace78/1, Scope78/1, Gain178/1, Gain177/1, Gain182/1  "y(k)=x1(k)"
  Sum80/1 -> Gain184/1, Sum78/3, To Workspace83/1, Scope83/1  "w2(k)"
  Gain181/1 -> Sum73/1
  Gain187/1 -> Sum78/1
  Gain179/1 -> Sum75/3
  Sum76/1 -> Gain181/1, To Workspace103/1, Gain186/1, Gain185/1, Gain179/1, Gain180/1  "u(k)"
  Gain191/1 -> Sum79/2
  Delay65/1 -> Sum79/1  "z1(k)"
  Sum78/1 -> Delay65/1  "z1(k+1)"
  Gain177/1 -> Sum74/1
  Gain178/1 -> Sum73/2
  Gain182/1 -> Sum75/1
  Gain189/1 -> Sum77/1
  Gain186/1 -> Sum77/2
  Sum77/1 -> Delay66/1  "z2(k+1)"
  Gain185/1 -> Sum78/2
  Gain188/1 -> Sum77/3
  Delay66/1 -> Sum80/1  "z2(k)"
  Sum87/1 -> To Workspace88/1, Scope88/1, Gain206/1, Gain207/1  "w1(k)"
  Gain193/1 -> Sum84/1
  Gain201/1 -> Sum84/3
  Gain200/1 -> Sum84/2
  Sum81/1 -> Delay67/1  "x3(k+1)"
  Delay68/1 -> To Workspace86/1, Scope86/1, Sum83/2  "x2(k)"
  Gain207/1 -> Sum86/4
  Sum82/1 -> Delay68/1  "x2(k+1)"
  Gain197/1 -> Sum82/3
  Sum83/1 -> Delay69/1  "x1(k+1)"
  Gain209/1 -> Sum88/2
  Delay67/1 -> To Workspace87/1, Scope87/1, Sum82/2  "x3(k)"
  Delay69/1 -> To Workspace85/1, Scope85/1, Gain209/1, Gain208/1, Gain205/1, Gain204/1, Gain193/1, To Workspace84/1, Scope84/1, Gain195/1, Gain194/1, Gain199/1  "y(k)=x1(k)"
  Sum88/1 -> Gain201/1, Sum86/3, To Workspace89/1, Scope89/1  "w2(k)"
  Gain198/1 -> Sum81/1
  Gain204/1 -> Sum86/1
  Gain196/1 -> Sum83/3
  Sum84/1 -> Gain198/1, To Workspace104/1, Scope104/1, Gain203/1, Gain202/1, Gain196/1, Gain197/1  "u(k)"
  Gain208/1 -> Gain200/1, Sum87/2
  Delay70/1 -> Sum87/1  "z1(k)"
  Sum86/1 -> Delay70/1  "z1(k+1)"
  Gain194/1 -> Sum82/1
  Gain195/1 -> Sum81/2
  Gain199/1 -> Sum83/1
  Gain206/1 -> Sum85/1
  Gain203/1 -> Sum85/2
  Sum85/1 -> Delay71/1  "z2(k+1)"
  Gain202/1 -> Sum86/2
  Gain205/1 -> Sum85/3
  Delay71/1 -> Sum88/1  "z2(k)"
  Sum95/1 -> To Workspace94/1, Scope94/1, Gain223/1, Gain224/1, Gain217/1  "w1(k)"
  Gain210/1 -> Sum92/1
  Gain218/1 -> Sum92/3
  Gain217/1 -> Sum92/2
  Sum89/1 -> Delay72/1  "x3(k+1)"
  Delay73/1 -> To Workspace92/1, Scope92/1, Sum91/2  "x2(k)"
  Gain224/1 -> Sum94/4
  Sum90/1 -> Delay73/1  "x2(k+1)"
  Gain214/1 -> Sum90/3
  Sum91/1 -> Delay74/1  "x1(k+1)"
  Gain226/1 -> Sum96/2
  Delay72/1 -> To Workspace93/1, Scope93/1, Sum90/2  "x3(k)"
  Delay74/1 -> To Workspace91/1, Scope91/1, Gain226/1, Gain225/1, Gain222/1, Gain221/1, Gain210/1, To Workspace90/1, Scope90/1, Gain212/1, Gain211/1, Gain216/1  "y(k)=x1(k)"
  Sum96/1 -> Gain218/1, Sum94/3, To Workspace95/1, Scope95/1  "w2(k)"
  Gain215/1 -> Sum89/1
  Gain221/1 -> Sum94/1
  Gain213/1 -> Sum91/3
  Sum92/1 -> Gain215/1, Scope105/1, To Workspace105/1, Gain220/1, Gain219/1, Gain213/1, Gain214/1  "u(k)"
  Gain225/1 -> Sum95/2
  Delay75/1 -> Sum95/1  "z1(k)"
  Sum94/1 -> Delay75/1  "z1(k+1)"
  Gain211/1 -> Sum90/1
  Gain212/1 -> Sum89/2
  Gain216/1 -> Sum91/1
  Gain223/1 -> Sum93/1
  Gain220/1 -> Sum93/2
  Sum93/1 -> Delay76/1  "z2(k+1)"
  Gain219/1 -> Sum94/2
  Gain222/1 -> Sum93/3
  Delay76/1 -> Sum96/1  "z2(k)"
  Sum103/1 -> Gain234/1, To Workspace100/1, Scope100/1, Gain240/1, Gain241/1  "w1(k)"
  Gain227/1 -> Sum100/1
  Gain235/1 -> Sum100/3
  Gain234/1 -> Sum100/2
  Sum97/1 -> Delay77/1  "x3(k+1)"
  Delay78/1 -> To Workspace98/1, Scope98/1, Sum99/2  "x2(k)"
  Gain241/1 -> Sum102/4
  Sum98/1 -> Delay78/1  "x2(k+1)"
  Gain231/1 -> Sum98/3
  Sum99/1 -> Delay79/1  "x1(k+1)"
  Gain243/1 -> Sum104/2
  Delay77/1 -> To Workspace99/1, Scope99/1, Sum98/2  "x3(k)"
  Delay79/1 -> To Workspace97/1, Scope97/1, Gain243/1, Gain242/1, Gain239/1, Gain238/1, Gain227/1, To Workspace96/1, Scope96/1, Gain229/1, Gain228/1, Gain233/1  "y(k)=x1(k)"
  Sum104/1 -> Gain235/1, Sum102/3, To Workspace101/1, Scope101/1  "w2(k)"
  Gain232/1 -> Sum97/1
  Gain238/1 -> Sum102/1
  Gain230/1 -> Sum99/3
  Gain242/1 -> Sum103/2
  Delay80/1 -> Sum103/1  "z1(k)"
  Sum102/1 -> Delay80/1  "z1(k+1)"
  Gain228/1 -> Sum98/1
  Gain229/1 -> Sum97/2
  Gain233/1 -> Sum99/1
  Gain240/1 -> Sum101/1
  Gain237/1 -> Sum101/2
  Sum101/1 -> Delay81/1  "z2(k+1)"
  Gain236/1 -> Sum102/2
  Gain239/1 -> Sum101/3
  Delay81/1 -> Sum104/1  "z2(k)"
  Sum100/1 -> Gain232/1, Scope106/1, To Workspace106/1, Gain237/1, Gain236/1, Gain230/1, Gain231/1  "u(k)"
  Delay83/1 -> Gain258/1, To Workspace108/1, Scope108/1, Gain256/1  "x3est(k)"
  Sum110/1 -> To Workspace110/1, Scope113/1, Sum111/1, Sum108/1  "u(k)"
  Gain258/1 -> Sum106/3
  Gain247/1 -> Sum109/2
  Gain256/1 -> Sum111/3
  Gain260/1 -> Sum105/2  "l3(y(k)-yest(k))"
  Gain254/1 -> Sum111/5
  Gain250/1 -> Sum109/3
  Delay86/1 -> Gain246/1, Gain253/1, To Workspace113/1, Scope112/1, Gain250/1  "x3(k) (z^-3)E(z)"
  Gain245/1 -> Sum109/1
  Gain253/1 -> Sum110/3  "-k3x3(k)"
  Sum109/1 -> To Workspace109/1, Sum107/2, Scope109/1  "y(k) Y(z)"
  Delay87/1 -> Gain254/1, Gain244/1, To Workspace114/1, Scope114/1, Sum112/1  "x1est(k)"
  Sum111/1 -> Delay87/1  "x1est(k+1)"
  Sum112/1 -> Delay82/1  "x2est(k+1)"
  Gain251/1 -> Sum110/1  "-k1x1(k)"
  Gain257/1 -> Sum106/2
  Gain244/1 -> Sum106/1
  Sum105/1 -> Delay83/1  "x3est(k+1)"
  Delay84/1 -> Gain249/1, Gain245/1, Delay85/1, Gain251/1, To Workspace111/1, Scope110/1  "x2(k+1)=x1(k) (z^-1)E(z)"
  Delay85/1 -> Gain252/1, To Workspace112/1, Scope111/1, Gain247/1, Delay86/1, Gain248/1  "x3(k+1)=x2(k) (z^-2)E(z)"
  Gain248/1 -> Sum108/2
  Gain261/1 -> Sum111/2  "l1(y(k)-yest(k))"
  Gain255/1 -> Sum111/4
  Gain246/1 -> Sum108/4
  Gain249/1 -> Sum108/3
  Delay82/1 -> Gain255/1, Gain257/1, To Workspace107/1, Scope107/1, Sum105/1  "x2est(k)"
  Sum107/1 -> Gain260/1, Gain259/1, Gain261/1  "(y(k)-yest(k))"
  Gain259/1 -> Sum112/2  "l2(y(k)-yest(k))"
  Sum106/1 -> Sum107/1  "yest(k)"
  Sum108/1 -> Delay84/1  "x1(k+1) E(z)"
  Gain252/1 -> Sum110/2  "-k2x2(k)"
